simulink model "Katex_FullCar_R2017b_V03"  (R2026a)
settings: Solver=ode1  StopTime=1000  FixedStep=Ts  EnableMultiTasking=on
PostLoadFcn:
  | , if any(exist('dsrtsu_mdlpostloadfcn', 'file') == [2, 3, 6]), try dsrtsu_mdlpostloadfcn('Execute', bdroot); catch fprintf('Error in PostLoadFcn (dsrtsu_mdlpostloadfcn) for model "%s":\n %s\n', bdroot, lasterr); end, end,
  | , if any(exist('dsrtsu_mdlpostloadfcn', 'file') ~= 0), dsrtsu_mdlpostloadfcn('Execute', bdroot); end,
InitFcn:
  | , if any(exist('rtifpga_mdlclblib', 'file') ~= 0), rtifpga_mdlclblib('Init', bdroot); end,
  | 
  | 
  | init
undefined symbols (not defined in the file): locklim_sus, roundN, Ts
libraries: sl_discontinuities x29, simulink_extras x26, simulink x22, mjLib x1
(part 10 of 10)

== matlab function Katex_FullCar_R2017b_V03/DGIST/_High_Level_Ctrl/Orientation_Vel_Ctrl/MATLAB Function ==
  data: RollRate_ref input; SusVel_ref output; PitchRate_ref input; RollRate_IMU_LPF input; PitchRate_IMU_LPF input; disturbance input; SusPos_act input; RobotWidth input; RobotLength input; SusLinkLength input; DOB_cutoff_freq input; Ts input; DOB_onoff input; z_vel_ref output; dhat_lpf output; z_vel_from_IMU output
function [SusVel_ref, z_vel_ref, dhat_lpf, z_vel_from_IMU] = ...
    Orientation_DOB_Discrete( ...
        RollRate_ref, PitchRate_ref, ...
        RollRate_IMU_LPF, PitchRate_IMU_LPF, ...
        disturbance, ...
        SusPos_act, RobotWidth, RobotLength, SusLinkLength, ...
        DOB_cutoff_freq, Ts, DOB_onoff)
%#codegen
% Discrete-time implementation of MuJoCo ori_DOB_run().
%
% Vector order: FL, FR, RL, RR
% Angle unit: rad
% Angular velocity unit: rad/s
% Length and vertical velocity units: m, m/s
%
% z_vel_control : command calculated before test disturbance [m/s]
% z_vel_ref     : command delivered to the plant after disturbance [m/s]
% SusVel_ref    : suspension load-side angular velocity command [rad/s]
% disturbance   : test disturbance added to the plant command [4x1, m/s]


% DOB LPF states: FL, FR, RL, RR
persistent dhat_input_old dhat_output_old

if isempty(dhat_input_old)
    dhat_input_old  = zeros(4,1);
    dhat_output_old = zeros(4,1);
end

% Fixed-size outputs for Simulink code generation
SusVel_ref     = zeros(4,1);
z_vel_ref      = zeros(4,1);
dhat_lpf       = zeros(4,1);
z_vel_from_IMU = zeros(4,1);

% =========================================================
% 1. Parameter validation
% =========================================================
if Ts <= 0 || RobotWidth < 0 || RobotLength <= 0 || ...
        SusLinkLength <= 0 || DOB_cutoff_freq <= 0
    return;
end

% =========================================================
% 2. Orientation Jacobian
% =========================================================
J_ori = zeros(4,2);

J_ori(1,1) =  RobotWidth/2.0 + SusLinkLength*cos(SusPos_act(1));
J_ori(1,2) = -RobotLength/2.0;

J_ori(2,1) = -(RobotWidth/2.0 + SusLinkLength*cos(SusPos_act(2)));
J_ori(2,2) = -RobotLength/2.0;

J_ori(3,1) =  RobotWidth/2.0 + SusLinkLength*cos(SusPos_act(3));
J_ori(3,2) =  RobotLength/2.0;

J_ori(4,1) = -(RobotWidth/2.0 + SusLinkLength*cos(SusPos_act(4)));
J_ori(4,2) =  RobotLength/2.0;

body_rate_ref = zeros(2,1);
body_rate_ref(1) = RollRate_ref;
body_rate_ref(2) = PitchRate_ref;

body_rate_IMU = zeros(2,1);
body_rate_IMU(1) = RollRate_IMU_LPF;
body_rate_IMU(2) = PitchRate_IMU_LPF;

% Nominal suspension vertical-velocity command
z_vel_nominal = J_ori * body_rate_ref;

% Measured body rates mapped to suspension vertical velocities
z_vel_from_IMU = J_ori * body_rate_IMU;

% =========================================================
% 3. DOB compensation
%    Previous LPF output is used to avoid an algebraic loop.
% =========================================================
if DOB_onoff ~= 0
    z_vel_control = z_vel_nominal - dhat_output_old;
else
    z_vel_control = z_vel_nominal;
end

% =========================================================
% 4. Disturbance estimation and discrete first-order LPF
%    The estimator remains active when DOB compensation is off.
% =========================================================
dhat_raw = z_vel_from_IMU - z_vel_control;
dhat_tau = 1.0/(2.0*pi*DOB_cutoff_freq);

for i = 1:4
    dhat_lpf(i) = ...
        (Ts*(dhat_raw(i) + dhat_input_old(i)) ...
        - (Ts - 2.0*dhat_tau)*dhat_output_old(i)) ...
        / (Ts + 2.0*dhat_tau);
end

dhat_input_old  = dhat_raw;
dhat_output_old = dhat_lpf;

% =========================================================
% 5. Test disturbance injection
% =========================================================
z_vel_ref = z_vel_control + disturbance;

% =========================================================
% 6. Vertical velocity -> suspension load-side joint velocity
%    MuJoCo ori_DOB_run(): q_dot = -z_dot/(L*cos(q))
% =========================================================
Denominator_threshold = 1.0e-6;

for i = 1:4
    denominator = SusLinkLength*cos(SusPos_act(i));

    if abs(denominator) < Denominator_threshold
        if denominator < 0
            denominator = -Denominator_threshold;
        else
            denominator = Denominator_threshold;
        end
    end
%부호 확인 필요
    SusVel_ref(i) = -z_vel_ref(i)/denominator;
end

end
